simulink model "AccPed_DrvDemStpLim"  (R2018a)
settings: configuration reference "cs_ert" (kept outside this file)
model workspace (MAT data in the model file):
  AccPed_DrvDemStpLim_DT = 10
settings Model: DataDictionary=AccPed_DrvDemStpLim.sldd  Creator=zhoutinglin  LastModifiedBy=zhoutinglin

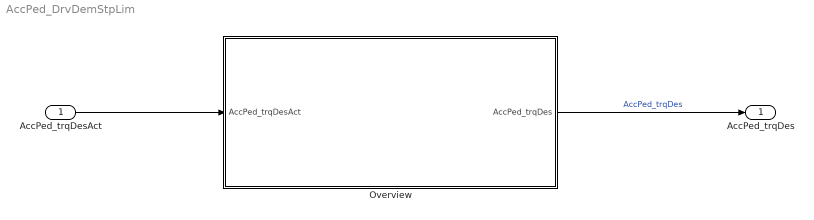
== system AccPed_DrvDemStpLim ==
  AccPed_trqDesAct : Inport  Description=driver torque raw of propulsion  OutMin=-3000  OutMax=3000  OutDataTypeStr=Torq  Unit=Nm  PortDimensions=[1 1]
  Overview : Subsystem
  AccPed_trqDes : Outport
  wires:
  AccPed_trqDesAct/1 -> Overview/1(AccPed_trqDesAct)
  Overview/1(AccPed_trqDes) -> AccPed_trqDes/1  "AccPed_trqDes"

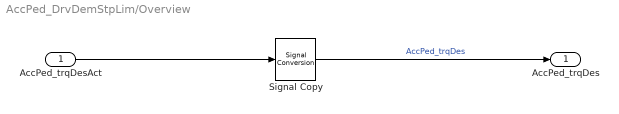
== system AccPed_DrvDemStpLim/Overview ==
  AccPed_trqDesAct : Inport  Tag=Nm
  Signal Copy : SignalConversion  OverrideOpt=off
  AccPed_trqDes : Outport  Tag=Nm
  wires:
  Signal Copy/1 -> AccPed_trqDes/1  "AccPed_trqDes"
  AccPed_trqDesAct/1 -> Signal Copy/1
